simulink model "autoMBD_example_PI_StructArg"  (R2020b)
settings: Solver=FixedStepAuto  StartTime=0.0  StopTime=10.0  FixedStep=0.001  RelTol=1e-3
undefined symbols (not defined in the file or in its folder): DiscIntNeverNeededParam
settings Model: Creator=k  LastModifiedBy=k
settings OptimizationCC: DefaultParameterBehavior=Inlined  EnhancedBackFolding=on  PassReuseOutputArgsAs=Individual arguments  ZeroExternalMemoryAtStartup=off  ZeroInternalMemoryAtStartup=off  OptimizeBlockOrder=speed  DifferentSizesBufferReuse=on  OptimizationCustomize=off  EfficientTunableParamExpr=on
settings DebuggingCC: ParameterTunabilityLossMsg=error
settings SFSimCC: MATLABDynamicMemAlloc=off
settings RTWCC: Description=Embedded Coder  SystemTargetFile=ert.tlc  GenCodeOnly=on  TemplateMakefile=ert_default_tmf
settings CodeAppCC: ForceParamTrailComments=on  IgnoreCustomStorageClasses=off  OperatorAnnotations=on  SimulinkDataObjDesc=on  SFDataObjDesc=on  InsertBlockDesc=on
settings ERTTargetCC: TargetLangStandard=C99 (ISO)  GenerateSampleERTMain=on  InlinedParameterPlacement=NonHierarchical  ERTCustomFileTemplate=example_file_process.tlc

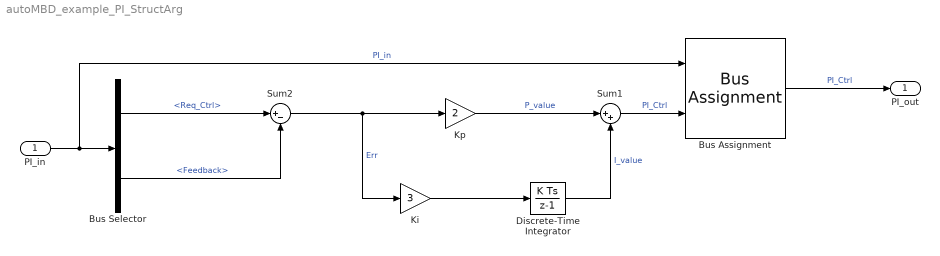
== system autoMBD_example_PI_StructArg ==
  PI_in : Inport  OutDataTypeStr=Bus: ctrlPI_struct
  Bus Assignment : BusAssignment  AssignedSignals=PI_Ctrl
  Bus Selector : BusSelector  OutputSignals=Req_Ctrl,Feedback
  Discrete-Time Integrator : DiscreteIntegrator  SampleTime=-1  ICPrevOutput=DiscIntNeverNeededParam  ICPrevScaledInput=DiscIntNeverNeededParam
  Ki : Gain  Gain=3
  Kp : Gain  Gain=2
  Sum1 : Sum  Inputs=|++
  Sum2 : Sum  Inputs=|+-
  PI_out : Outport  OutDataTypeStr=Bus: ctrlPI_struct
  wires:
  Sum1/1 -> Bus Assignment/2  "PI_Ctrl"
  Bus Selector/2 -> Sum2/2  "<Feedback>"
  Bus Selector/1 -> Sum2/1  "<Req_Ctrl>"
  Sum2/1 -> Ki/1, Kp/1  "Err"
  Kp/1 -> Sum1/1  "P_value"
  Ki/1 -> Discrete-Time Integrator/1
  Discrete-Time Integrator/1 -> Sum1/2  "I_value"
  PI_in/1 -> Bus Assignment/1, Bus Selector/1  "PI_in"
  Bus Assignment/1 -> PI_out/1  "PI_Ctrl"
